simulink model "PCM"  (R2018a)
settings: Solver=VariableStepAuto  StartTime=0.0  StopTime=50.0  RelTol=1e-3
libraries: commsrccod2 x2, dspquant2 x2, dsparch4 x1, simulink x1
settings Model: Creator=mengmeng  LastModifiedBy=mengmeng

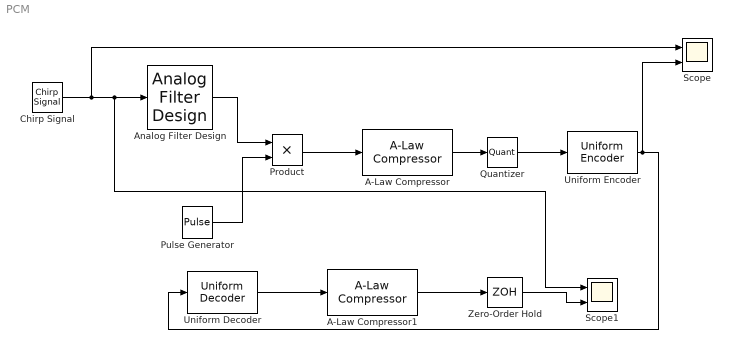
== system PCM ==
  A-Law Compressor : commsrccod2/A-Law Compressor  A=87.6  V=1
      settings: SourceProductName=Communications System Toolbox  SourceProductBaseCode=CM
  A-Law Compressor1 : commsrccod2/A-Law Compressor  A=87.6  V=1
      settings: SourceProductName=Communications System Toolbox  SourceProductBaseCode=CM
  Analog Filter Design : dsparch4/Analog Filter Design  method=Butterworth  filttype=Lowpass  N=8  Wlo=30  Whi=80  Rp=2  Rs=40
  Chirp Signal : simulink/Sources/Chirp Signal  f1=0.1  T=100  f2=1
  Product : Product
  Pulse Generator : DiscretePulseGenerator  PulseType=Time based  PulseWidth=50
  Quantizer : Quantizer
  Scope : Scope  NumInputPorts=2
  Scope1 : Scope  NumInputPorts=2
  Uniform Decoder : dspquant2/Uniform Decoder  peak=1  bits=3  overflowMode=Saturate  otype=Double
      settings: SourceProductName=DSP System Toolbox  SourceProductBaseCode=DS
  Uniform Encoder : dspquant2/Uniform Encoder  peak=1  bits=8  otype=Unsigned integer
      settings: SourceProductName=DSP System Toolbox
  Zero-Order Hold : ZeroOrderHold  SampleTime=-1
  wires:
  Chirp Signal/1 -> Scope/1, Scope1/1, Analog Filter Design/1
  Analog Filter Design/1 -> Product/1
  Pulse Generator/1 -> Product/2
  Product/1 -> A-Law Compressor/1
  A-Law Compressor/1 -> Quantizer/1
  Quantizer/1 -> Uniform Encoder/1
  Uniform Encoder/1 -> Scope/2, Uniform Decoder/1
  Uniform Decoder/1 -> A-Law Compressor1/1
  A-Law Compressor1/1 -> Zero-Order Hold/1
  Zero-Order Hold/1 -> Scope1/2
